simulink model "NichtLinearesModell"  (R2021b)
settings: Solver=ode4  StartTime=0.0  StopTime=250  FixedStep=0.02  RelTol=1e-3
undefined symbols (not defined in the file): AC, BFZ, c, ENV, input_height, input_speed, k_lag, k_p, NickD
settings Model: Creator=falcon  LastModifiedBy=jonih
settings DebuggingCC: UnderSpecifiedDimensionMsg=warning

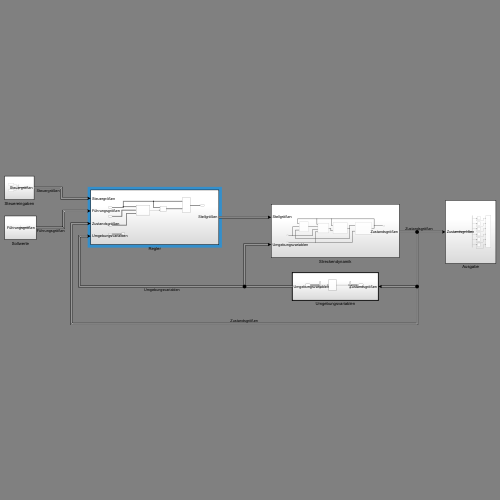
[thumbnail: Simulink's stored preview of the top-level diagram]
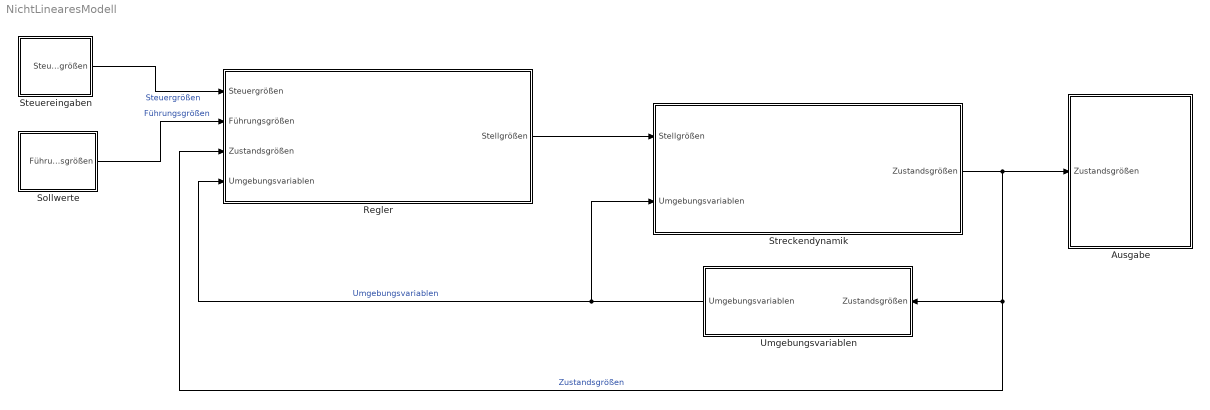
== system NichtLinearesModell ==
  Ausgabe : Subsystem
  Regler : Subsystem
  Sollwerte : Subsystem
  Steuereingaben : Subsystem
  Streckendynamik : Subsystem
  Umgebungsvariablen : Subsystem  TreatAsAtomicUnit=on
  wires:
  Streckendynamik/1(Zustandsgrößen) -> Umgebungsvariablen/1(Zustandsgrößen), Regler/3(Zustandsgrößen), Ausgabe/1(Zustandsgrößen)  "Zustandsgrößen"
  Umgebungsvariablen/1(Umgebungsvariablen) -> Streckendynamik/2(Umgebungsvariablen), Regler/4(Umgebungsvariablen)  "Umgebungsvariablen"
  Sollwerte/1(Führungsgrößen) -> Regler/2(Führungsgrößen)  "Führungsgrößen"
  Steuereingaben/1(Steuergrößen) -> Regler/1(Steuergrößen)  "Steuergrößen"
  Regler/1(Stellgrößen) -> Streckendynamik/1(Stellgrößen)

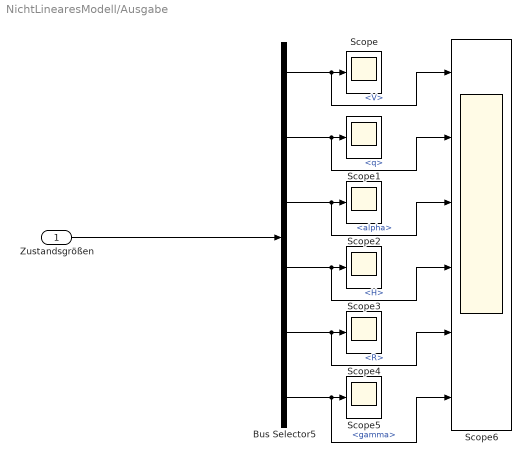
== system NichtLinearesModell/Ausgabe ==
  Zustandsgrößen : Inport
  Bus Selector5 : BusSelector  OutputSignals=V,q,alpha,H,R,gamma
  Scope{,1..5} (6 alike) : Scope
  Scope6 : Scope  NumInputPorts=6
  wires:
  Bus Selector5/4 -> Scope6/4, Scope3/1  "<H>"
  Zustandsgrößen/1 -> Bus Selector5/1
  Bus Selector5/3 -> Scope6/3, Scope2/1  "<alpha>"
  Bus Selector5/6 -> Scope6/6, Scope5/1  "<gamma>"
  Bus Selector5/2 -> Scope6/2, Scope1/1  "<q>"
  Bus Selector5/5 -> Scope6/5, Scope4/1  "<R>"
  Bus Selector5/1 -> Scope6/1, Scope/1  "<V>"

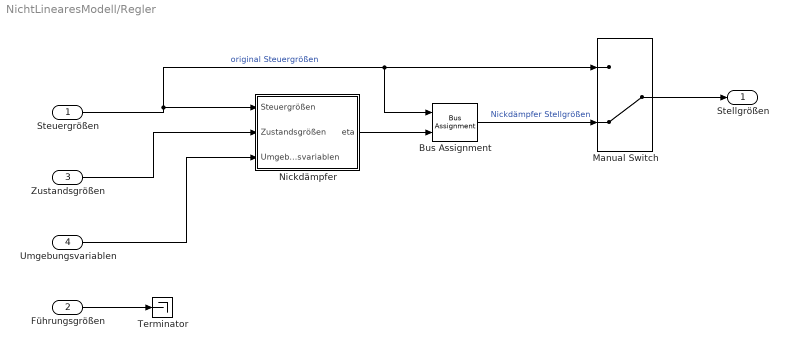
== system NichtLinearesModell/Regler ==
  Steuergrößen : Inport
  Führungsgrößen : Inport  Port=2
  Zustandsgrößen : Inport  Port=3
  Umgebungsvariablen : Inport  Port=4
  Bus Assignment : BusAssignment  AssignedSignals=eta
  Manual Switch : ManualSwitch  CurrentSetting=0
  Nickdämpfer : Subsystem
  Terminator : Terminator
  Stellgrößen : Outport
  wires:
  Steuergrößen/1 -> Nickdämpfer/1(Steuergrößen), Bus Assignment/1, Manual Switch/1  "original Steuergrößen"
  Zustandsgrößen/1 -> Nickdämpfer/2(Zustandsgrößen)
  Nickdämpfer/1(eta) -> Bus Assignment/2
  Führungsgrößen/1 -> Terminator/1
  Bus Assignment/1 -> Manual Switch/2  "Nickdämpfer Stellgrößen"
  Manual Switch/1 -> Stellgrößen/1
  Umgebungsvariablen/1 -> Nickdämpfer/3(Umgebungsvariablen)

== system NichtLinearesModell/Sollwerte ==
  Bus Creator : BusCreator  Inputs=1
  Führungsgrößendummy : Constant  Value=0
  Führungsgrößen : Outport
  wires:
  Führungsgrößendummy/1 -> Bus Creator/1
  Bus Creator/1 -> Führungsgrößen/1  "Führungsgrößen"

== system NichtLinearesModell/Steuereingaben ==
  Bus Creator2 : BusCreator  Inputs=2
  Höhenruderausschlag : Constant  Value=BFZ(8).eta
  Schubdrosselstellung : Constant  Value=BFZ(8).delta
  Steuergrößen : Outport
  wires:
  Höhenruderausschlag/1 -> Bus Creator2/1  "eta"
  Bus Creator2/1 -> Steuergrößen/1  "Steuergrößen"
  Schubdrosselstellung/1 -> Bus Creator2/2  "delta"

== system NichtLinearesModell/Streckendynamik ==
  Stellgrößen : Inport
  Umgebungsvariablen : Inport  Port=2
  Beiwerteberechnung : Subsystem
  Integration : Subsystem
  Kräfte und Momente : Subsystem
  zeitliche Änderung der Zustandsgrößen : Subsystem
  Zustandsgrößen : Outport
  wires:
  Beiwerteberechnung/1(Beiwerte) -> Kräfte und Momente/2(Beiwerte)  "Beiwerte"
  Stellgrößen/1 -> Beiwerteberechnung/2(Steuergrößen), Kräfte und Momente/3(Steuergrößen)  "Stellgrößen"
  Kräfte und Momente/1(Kräfte & Momente) -> zeitliche Änderung der Zustandsgrößen/2(Kräfte & Momente)
  Integration/1(Zustandsgrößen) -> Beiwerteberechnung/1(Zustandsgrößen), Kräfte und Momente/1(Zustandsgrößen), zeitliche Änderung der Zustandsgrößen/1(Zustandsgrößen), Zustandsgrößen/1  "Zustandsgrößen"
  zeitliche Änderung der Zustandsgrößen/1(Änderung der Zustandsgrößen) -> Integration/1(zeitl. Änderung d. Zustandsgrößen), Beiwerteberechnung/3(Änderung der Zustandsgrößen)  "zeitl. Änderung der Zustandsgrößen"
  Umgebungsvariablen/1 -> Kräfte und Momente/4(Umgebungsvariablen), Integration/2(Umgebungsvariablen)  "Umgebungsvariablen"

== system NichtLinearesModell/Umgebungsvariablen ==
  Zustandsgrößen : Inport
  Bus Creator : BusCreator  Inputs=1
  Bus Selector4 : BusSelector  OutputSignals=H
  rho_Berechnung : Subsystem
  Umgebungsvariablen : Outport
  wires:
  Bus Selector4/1 -> rho_Berechnung/1(H)  "<H>"
  rho_Berechnung/1(rho) -> Bus Creator/1  "rho"
  Bus Creator/1 -> Umgebungsvariablen/1
  Zustandsgrößen/1 -> Bus Selector4/1

== system NichtLinearesModell/Regler/Nickdämpfer ==
  Steuergrößen : Inport
  Zustandsgrößen : Inport  Port=2
  Umgebungsvariablen : Inport  Port=3
  Bus Selector : BusSelector  OutputSignals=eta
  Lag-Filter Rückführung : Subsystem
  Manual Switch : ManualSwitch
  Proportionalrückführung : Subsystem
  Sum : Sum  Inputs=+-|
  eta : Outport
  wires:
  Sum/1 -> eta/1  "eta"
  Lag-Filter Rückführung/1(η) -> Manual Switch/1
  Manual Switch/1 -> Sum/2
  Steuergrößen/1 -> Bus Selector/1
  Bus Selector/1 -> Sum/1  "<eta>"
  Proportionalrückführung/1(η) -> Manual Switch/2
  Zustandsgrößen/1 -> Lag-Filter Rückführung/1(Zustandsgrößen), Proportionalrückführung/1(Zustandsgrößen)
  Umgebungsvariablen/1 -> Lag-Filter Rückführung/2(Umgebungsvariablen), Proportionalrückführung/2(Umgebungsvariablen)

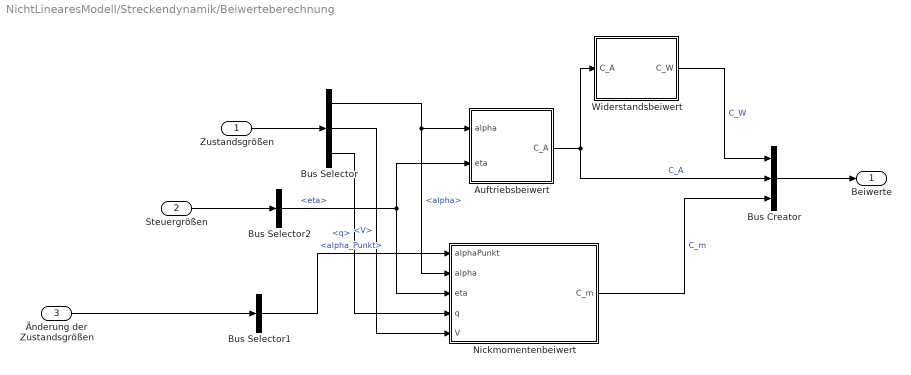
== system NichtLinearesModell/Streckendynamik/Beiwerteberechnung ==
  Zustandsgrößen : Inport
  Steuergrößen : Inport  Port=2
  Änderung der Zustandsgrößen : Inport  Port=3
  Auftriebsbeiwert : Subsystem
  Bus Creator : BusCreator  Inputs=3
  Bus Selector : BusSelector  OutputSignals=alpha,V,q
  Bus Selector1 : BusSelector  OutputSignals=alpha_Punkt
  Bus Selector2 : BusSelector  OutputSignals=eta
  Nickmomentenbeiwert : Subsystem
  Widerstandsbeiwert : Subsystem
  Beiwerte : Outport
  wires:
  Nickmomentenbeiwert/1(C_m) -> Bus Creator/3  "C_m"
  Auftriebsbeiwert/1(C_A) -> Bus Creator/2, Widerstandsbeiwert/1(C_A)  "C_A"
  Bus Selector/1 -> Auftriebsbeiwert/1(alpha), Nickmomentenbeiwert/2(alpha)  "<alpha>"
  Bus Creator/1 -> Beiwerte/1
  Widerstandsbeiwert/1(C_W) -> Bus Creator/1  "C_W"
  Zustandsgrößen/1 -> Bus Selector/1
  Änderung der Zustandsgrößen/1 -> Bus Selector1/1
  Bus Selector1/1 -> Nickmomentenbeiwert/1(alphaPunkt)  "<alpha_Punkt>"
  Bus Selector/2 -> Nickmomentenbeiwert/5(V)  "<V>"
  Bus Selector/3 -> Nickmomentenbeiwert/4(q)  "<q>"
  Steuergrößen/1 -> Bus Selector2/1
  Bus Selector2/1 -> Nickmomentenbeiwert/3(eta), Auftriebsbeiwert/2(eta)  "<eta>"

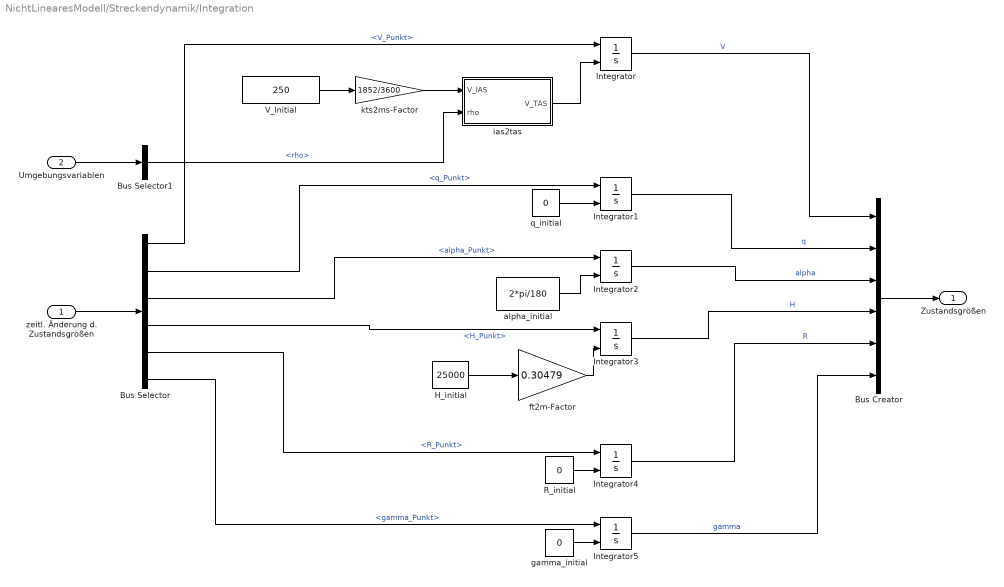
== system NichtLinearesModell/Streckendynamik/Integration ==
  zeitl. Änderung d. Zustandsgrößen : Inport
  Umgebungsvariablen : Inport  Port=2
  Bus Creator : BusCreator  Inputs=6
  Bus Selector : BusSelector  OutputSignals=V_Punkt,q_Punkt,alpha_Punkt,H_Punkt,R_Punkt,gamma_Punkt
  Bus Selector1 : BusSelector  OutputSignals=rho
  H_initial : Constant  Value=25000
  Integrator{,1..5} (6 alike) : Integrator  InitialConditionSource=external
  R_initial : Constant  Value=0
  V_Initial : Constant  Value=250
  alpha_initial : Constant  Value=2*pi/180
  ft2m-Factor : Gain  Gain=0.30479
  gamma_initial : Constant  Value=0
  ias2tas : Subsystem
  kts2ms-Factor : Gain  Gain=1852/3600
  q_initial : Constant  Value=0
  Zustandsgrößen : Outport
  wires:
  Bus Selector/5 -> Integrator4/1  "<R_Punkt>"
  gamma_initial/1 -> Integrator5/2
  Bus Selector/3 -> Integrator2/1  "<alpha_Punkt>"
  Integrator2/1 -> Bus Creator/3  "alpha"
  alpha_initial/1 -> Integrator2/2
  Integrator1/1 -> Bus Creator/2  "q"
  Integrator4/1 -> Bus Creator/5  "R"
  Integrator3/1 -> Bus Creator/4  "H"
  Integrator5/1 -> Bus Creator/6  "gamma"
  ias2tas/1(V_TAS) -> Integrator/2
  R_initial/1 -> Integrator4/2
  q_initial/1 -> Integrator1/2
  Bus Selector/6 -> Integrator5/1  "<gamma_Punkt>"
  Bus Selector/2 -> Integrator1/1  "<q_Punkt>"
  Bus Selector/4 -> Integrator3/1  "<H_Punkt>"
  Integrator/1 -> Bus Creator/1  "V"
  Bus Selector/1 -> Integrator/1  "<V_Punkt>"
  V_Initial/1 -> kts2ms-Factor/1
  kts2ms-Factor/1 -> ias2tas/1(V_IAS)
  Bus Selector1/1 -> ias2tas/2(rho)  "<rho>"
  H_initial/1 -> ft2m-Factor/1
  ft2m-Factor/1 -> Integrator3/2
  Bus Creator/1 -> Zustandsgrößen/1
  zeitl. Änderung d. Zustandsgrößen/1 -> Bus Selector/1
  Umgebungsvariablen/1 -> Bus Selector1/1

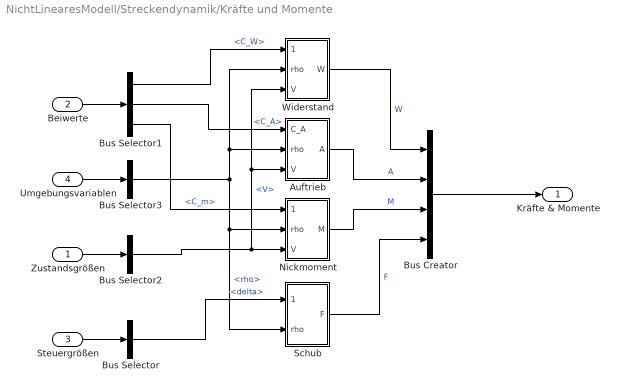
== system NichtLinearesModell/Streckendynamik/Kräfte und Momente ==
  Zustandsgrößen : Inport
  Beiwerte : Inport  Port=2
  Steuergrößen : Inport  Port=3
  Umgebungsvariablen : Inport  Port=4
  Auftrieb : Subsystem
  Bus Creator : BusCreator  Inputs=4
  Bus Selector : BusSelector  OutputSignals=delta
  Bus Selector1 : BusSelector  OutputSignals=C_W,C_A,C_m
  Bus Selector2 : BusSelector  OutputSignals=V
  Bus Selector3 : BusSelector  OutputSignals=rho
  Nickmoment : Subsystem
  Schub : Subsystem
  Widerstand : Subsystem
  Kräfte & Momente : Outport
  wires:
  Widerstand/1(W) -> Bus Creator/1  "W"
  Auftrieb/1(A) -> Bus Creator/2  "A"
  Nickmoment/1(M) -> Bus Creator/3  "M"
  Schub/1(F) -> Bus Creator/4  "F"
  Bus Creator/1 -> Kräfte & Momente/1
  Beiwerte/1 -> Bus Selector1/1
  Zustandsgrößen/1 -> Bus Selector2/1
  Steuergrößen/1 -> Bus Selector/1
  Bus Selector/1 -> Schub/1(delta)  "<delta>"
  Bus Selector1/2 -> Auftrieb/1(C_A)  "<C_A>"
  Bus Selector1/1 -> Widerstand/1(C_W)  "<C_W>"
  Bus Selector1/3 -> Nickmoment/1(C_m)  "<C_m>"
  Umgebungsvariablen/1 -> Bus Selector3/1
  Bus Selector3/1 -> Nickmoment/2(rho), Schub/2(rho), Auftrieb/2(rho), Widerstand/2(rho)  "<rho>"
  Bus Selector2/1 -> Nickmoment/3(V), Auftrieb/3(V), Widerstand/3(V)  "<V>"

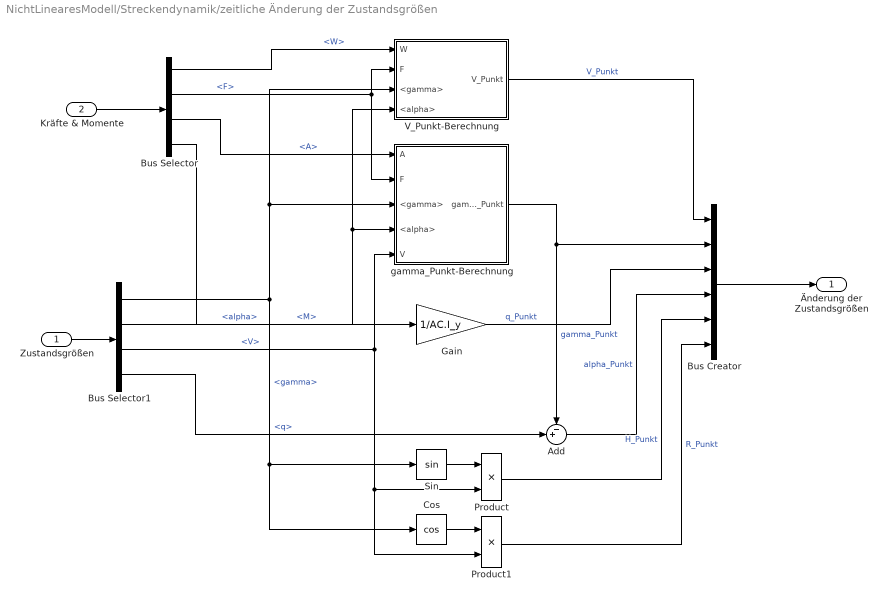
== system NichtLinearesModell/Streckendynamik/zeitliche Änderung der Zustandsgrößen ==
  Zustandsgrößen : Inport
  Kräfte & Momente : Inport  Port=2
  Add : Sum  Inputs=-+|
  Bus Creator : BusCreator  Inputs=6
  Bus Selector : BusSelector  OutputSignals=W,F,A,M
  Bus Selector1 : BusSelector  OutputSignals=gamma,alpha,V,q
  Cos : Trigonometry  Operator=cos
  Gain : Gain  Gain=1/AC.I_y
  Product : Product
  Product1 : Product
  Sin : Trigonometry
  V_Punkt-Berechnung : Subsystem
  gamma_Punkt-Berechnung : Subsystem
  Änderung der Zustandsgrößen : Outport
  wires:
  V_Punkt-Berechnung/1(V_Punkt) -> Bus Creator/1  "V_Punkt"
  Sin/1 -> Product/1
  Add/1 -> Bus Creator/4  "alpha_Punkt"
  Bus Selector/3 -> gamma_Punkt-Berechnung/1(A)  "<A>"
  gamma_Punkt-Berechnung/1(gamma_Punkt) -> Bus Creator/2, Add/1  "gamma_Punkt"
  Gain/1 -> Bus Creator/3  "q_Punkt"
  Bus Selector/4 -> Gain/1  "<M>"
  Cos/1 -> Product1/1
  Bus Selector/1 -> V_Punkt-Berechnung/1(W)  "<W>"
  Bus Selector1/2 -> gamma_Punkt-Berechnung/4(<alpha>), V_Punkt-Berechnung/4(<alpha>)  "<alpha>"
  Product/1 -> Bus Creator/5  "H_Punkt"
  Bus Selector1/1 -> Sin/1, Cos/1, V_Punkt-Berechnung/3(<gamma>), gamma_Punkt-Berechnung/3(<gamma>)  "<gamma>"
  Bus Selector1/3 -> Product1/2, Product/2, gamma_Punkt-Berechnung/5(V)  "<V>"
  Product1/1 -> Bus Creator/6  "R_Punkt"
  Bus Selector/2 -> gamma_Punkt-Berechnung/2(F), V_Punkt-Berechnung/2(F)  "<F>"
  Bus Selector1/4 -> Add/2  "<q>"
  Zustandsgrößen/1 -> Bus Selector1/1
  Kräfte & Momente/1 -> Bus Selector/1
  Bus Creator/1 -> Änderung der Zustandsgrößen/1

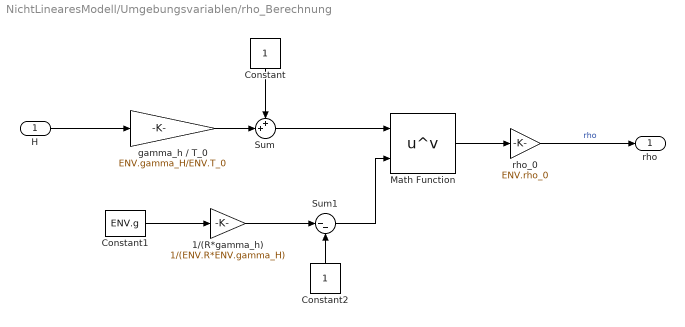
== system NichtLinearesModell/Umgebungsvariablen/rho_Berechnung ==
  H : Inport
  1/(R*gamma_h) : Gain  Gain=1/(ENV.R*ENV.gamma_H)
  Constant : Constant
  Constant1 : Constant  Value=ENV.g
  Constant2 : Constant
  Math Function : Math  Operator=pow  SaturateOnIntegerOverflow=on
  Sum : Sum  Inputs=++|
  Sum1 : Sum  Inputs=|--
  gamma_h / T_0 : Gain  Gain=ENV.gamma_H/ENV.T_0
  rho_0 : Gain  Gain=ENV.rho_0
  rho : Outport
  wires:
  1/(R*gamma_h)/1 -> Sum1/1
  gamma_h / T_0/1 -> Sum/2
  Constant1/1 -> 1/(R*gamma_h)/1
  Sum/1 -> Math Function/1
  H/1 -> gamma_h / T_0/1
  Sum1/1 -> Math Function/2
  rho_0/1 -> rho/1  "rho"
  Constant2/1 -> Sum1/2
  Math Function/1 -> rho_0/1
  Constant/1 -> Sum/1

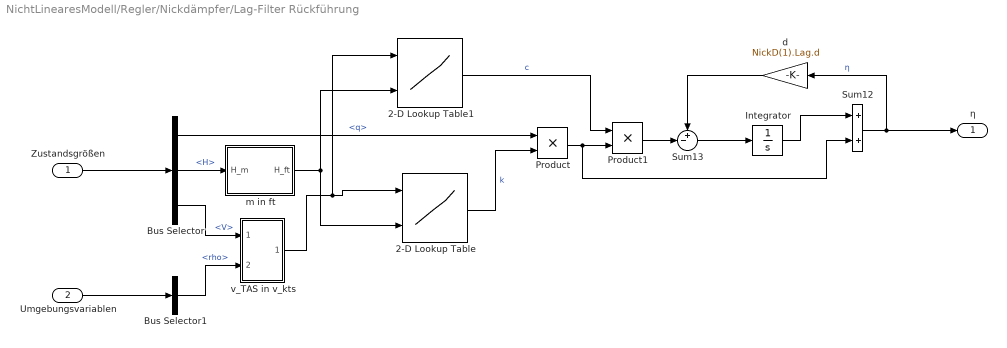
== system NichtLinearesModell/Regler/Nickdämpfer/Lag-Filter Rückführung ==
  Zustandsgrößen : Inport
  Umgebungsvariablen : Inport  Port=2
  2-D Lookup Table : Lookup_n-D  BreakpointsForDimension1=input_speed  BreakpointsForDimension2=input_height  Table=reshape(k_lag,[length(input_speed),length(input_height)])  InternalRulePriority=Speed  RndMeth=Simplest  InputSameDT=on
      settings: InputPortMap=u0,u1
  2-D Lookup Table1 : Lookup_n-D  BreakpointsForDimension1=input_speed  BreakpointsForDimension2=input_height  Table=reshape(c,[length(input_speed),length(input_height)])  InternalRulePriority=Speed  RndMeth=Simplest  InputSameDT=on
      settings: InputPortMap=u0,u1
  Bus Selector : BusSelector  OutputSignals=q,H,V
  Bus Selector1 : BusSelector  OutputSignals=rho
  Integrator : Integrator
  Product : Product
  Product1 : Product
  Sum12 : Sum
  Sum13 : Sum  Inputs=+-|
  d : Gain  Gain=NickD(1).Lag.d
  m in ft : Subsystem
  v_TAS in v_kts : Subsystem
  η : Outport
  wires:
  d/1 -> Sum13/1
  Sum13/1 -> Integrator/1
  Sum12/1 -> η/1, d/1  "η"
  Integrator/1 -> Sum12/1
  Product1/1 -> Sum13/2
  Zustandsgrößen/1 -> Bus Selector/1
  Bus Selector/1 -> Product/1  "<q>"
  Product/1 -> Product1/2, Sum12/2
  Bus Selector/3 -> v_TAS in v_kts/1(V_TAS)  "<V>"
  Umgebungsvariablen/1 -> Bus Selector1/1
  Bus Selector1/1 -> v_TAS in v_kts/2(rho)  "<rho>"
  Bus Selector/2 -> m in ft/1(H_m)  "<H>"
  2-D Lookup Table1/1 -> Product1/1  "c"
  2-D Lookup Table/1 -> Product/2  "k"
  m in ft/1(H_ft) -> 2-D Lookup Table/2, 2-D Lookup Table1/2
  v_TAS in v_kts/1(v_kts) -> 2-D Lookup Table1/1, 2-D Lookup Table/1

== system NichtLinearesModell/Regler/Nickdämpfer/Proportionalrückführung ==
  Zustandsgrößen : Inport
  Umgebungsvariablen : Inport  Port=2
  2-D Lookup Table : Lookup_n-D  BreakpointsForDimension1=input_speed  BreakpointsForDimension2=input_height  Table=reshape(k_p,[length(input_speed),length(input_height)])  InternalRulePriority=Speed  RndMeth=Simplest  InputSameDT=on
      settings: InputPortMap=u0,u1
  Bus Selector : BusSelector  OutputSignals=q,V,H
  Bus Selector2 : BusSelector  OutputSignals=rho
  Product : Product
  m in ft : Subsystem
  v_TAS in v_kts : Subsystem
  η : Outport
  wires:
  Product/1 -> η/1  "eta"
  Zustandsgrößen/1 -> Bus Selector/1
  Bus Selector/1 -> Product/1  "<q>"
  2-D Lookup Table/1 -> Product/2  "k_p"
  Umgebungsvariablen/1 -> Bus Selector2/1
  Bus Selector2/1 -> v_TAS in v_kts/2(rho)  "<rho>"
  Bus Selector/3 -> m in ft/1(H_m)  "<H>"
  Bus Selector/2 -> v_TAS in v_kts/1(V_TAS)  "<V>"
  m in ft/1(H_ft) -> 2-D Lookup Table/2
  v_TAS in v_kts/1(v_kts) -> 2-D Lookup Table/1

== system NichtLinearesModell/Streckendynamik/Beiwerteberechnung/Auftriebsbeiwert ==
  alpha : Inport
  eta : Inport  Port=2
  Constant1 : Constant  Value=AC.C_A_Alpha0Eta0
  Gain : Gain  Gain=AC.C_A_Eta
  Gain2 : Gain  Gain=AC.C_A_Alpha
  Sum : Sum  Inputs=+++
  C_A : Outport
  wires:
  Constant1/1 -> Sum/1
  Gain2/1 -> Sum/2
  eta/1 -> Gain/1
  Gain/1 -> Sum/3
  alpha/1 -> Gain2/1
  Sum/1 -> C_A/1  "C_A"

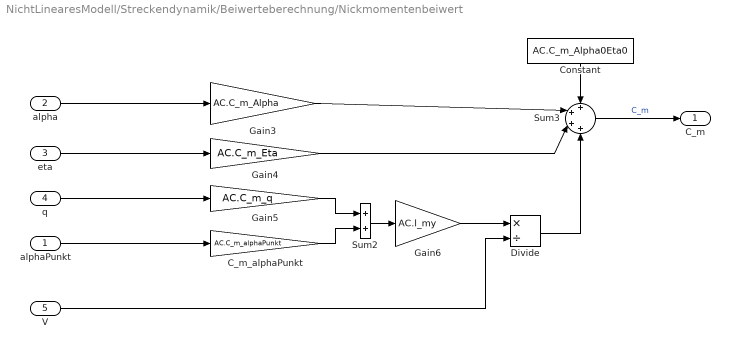
== system NichtLinearesModell/Streckendynamik/Beiwerteberechnung/Nickmomentenbeiwert ==
  alphaPunkt : Inport
  alpha : Inport  Port=2
  eta : Inport  Port=3
  q : Inport  Port=4
  V : Inport  Port=5
  C_m_alphaPunkt : Gain  Gain=AC.C_m_alphaPunkt
  Constant : Constant  Value=AC.C_m_Alpha0Eta0
  Divide : Product  Inputs=*/
  Gain3 : Gain  Gain=AC.C_m_Alpha
  Gain4 : Gain  Gain=AC.C_m_Eta
  Gain5 : Gain  Gain=AC.C_m_q
  Gain6 : Gain  Gain=AC.l_my
  Sum2 : Sum
  Sum3 : Sum  Inputs=++++
  C_m : Outport
  wires:
  Gain3/1 -> Sum3/2
  Divide/1 -> Sum3/4
  V/1 -> Divide/2
  C_m_alphaPunkt/1 -> Sum2/2
  Gain4/1 -> Sum3/3
  q/1 -> Gain5/1
  Constant/1 -> Sum3/1
  Gain6/1 -> Divide/1
  Gain5/1 -> Sum2/1
  alpha/1 -> Gain3/1
  Sum2/1 -> Gain6/1
  Sum3/1 -> C_m/1  "C_m"
  eta/1 -> Gain4/1
  alphaPunkt/1 -> C_m_alphaPunkt/1

== system NichtLinearesModell/Streckendynamik/Beiwerteberechnung/Widerstandsbeiwert ==
  C_A : Inport
  Constant2 : Constant  Value=AC.C_W0
  Gain1 : Gain  Gain=AC.k
  Square : Math  Operator=square  SaturateOnIntegerOverflow=on
  Sum1 : Sum  Inputs=|++
  C_W : Outport
  wires:
  Constant2/1 -> Sum1/1
  Sum1/1 -> C_W/1  "C_W"
  Square/1 -> Gain1/1
  C_A/1 -> Square/1
  Gain1/1 -> Sum1/2

== system NichtLinearesModell/Streckendynamik/Integration/ias2tas ==
  V_IAS : Inport
  rho : Inport  Port=2
  Constant : Constant  Value=1.225
  Divide : Product  Inputs=*/
  Product : Product
  Sqrt : Sqrt  SaturateOnIntegerOverflow=on
  V_TAS : Outport
  wires:
  Product/1 -> V_TAS/1
  V_IAS/1 -> Product/1
  Constant/1 -> Divide/1
  rho/1 -> Divide/2
  Divide/1 -> Sqrt/1
  Sqrt/1 -> Product/2

== system NichtLinearesModell/Streckendynamik/Kräfte und Momente/Auftrieb ==
  C_A : Inport
  rho : Inport  Port=2
  V : Inport  Port=3
  Gain : Gain  Gain=0.5
  Gain1 : Gain  Gain=AC.S
  Product : Product  Inputs=3
  Square : Math  Operator=square  SaturateOnIntegerOverflow=on
  A : Outport
  wires:
  rho/1 -> Gain/1
  Square/1 -> Product/3
  Product/1 -> Gain1/1
  Gain1/1 -> A/1  "A"
  V/1 -> Square/1
  Gain/1 -> Product/2
  C_A/1 -> Product/1

== system NichtLinearesModell/Streckendynamik/Kräfte und Momente/Nickmoment ==
  C_m : Inport
  rho : Inport  Port=2
  V : Inport  Port=3
  Gain : Gain  Gain=0.5
  Gain1 : Gain  Gain=AC.S
  Gain2 : Gain  Gain=AC.l_my
  Product : Product  Inputs=3
  Square : Math  Operator=square  SaturateOnIntegerOverflow=on
  M : Outport
  wires:
  rho/1 -> Gain/1
  Square/1 -> Product/3
  Product/1 -> Gain1/1
  Gain1/1 -> Gain2/1
  V/1 -> Square/1
  Gain/1 -> Product/2
  C_m/1 -> Product/1
  Gain2/1 -> M/1

== system NichtLinearesModell/Streckendynamik/Kräfte und Momente/Schub ==
  delta : Inport
  rho : Inport  Port=2
  Constant : Constant  Value=AC.n_rho
  Gain : Gain  Gain=AC.F_TBPmax
  Math Function : Math  Operator=pow  SaturateOnIntegerOverflow=on
  Multiply : Gain  Gain=1/AC.rho_TBP
  Product : Product
  F : Outport
  wires:
  rho/1 -> Multiply/1
  Constant/1 -> Math Function/2
  Product/1 -> F/1  "F"
  Math Function/1 -> Product/2
  Gain/1 -> Product/1
  Multiply/1 -> Math Function/1
  delta/1 -> Gain/1

== system NichtLinearesModell/Streckendynamik/Kräfte und Momente/Widerstand ==
  C_W : Inport
  rho : Inport  Port=2
  V : Inport  Port=3
  Gain : Gain  Gain=0.5
  Gain1 : Gain  Gain=AC.S
  Product : Product  Inputs=3
  Square : Math  Operator=square  SaturateOnIntegerOverflow=on
  W : Outport
  wires:
  rho/1 -> Gain/1
  Square/1 -> Product/3
  Product/1 -> Gain1/1
  Gain1/1 -> W/1  "W"
  V/1 -> Square/1
  Gain/1 -> Product/2
  C_W/1 -> Product/1

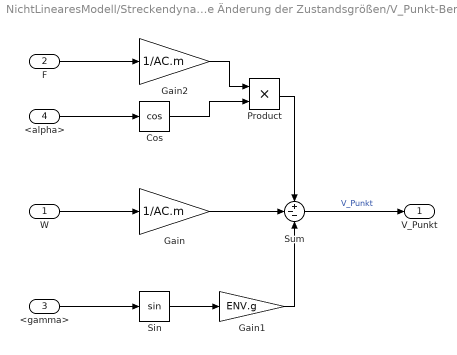
== system NichtLinearesModell/Streckendynamik/zeitliche Änderung der Zustandsgrößen/V_Punkt-Berechnung ==
  W : Inport
  F : Inport  Port=2
  <gamma> : Inport  Port=3
  <alpha> : Inport  Port=4
  Cos : Trigonometry  Operator=cos
  Gain : Gain  Gain=1/AC.m
  Gain1 : Gain  Gain=ENV.g
  Gain2 : Gain  Gain=1/AC.m
  Product : Product
  Sin : Trigonometry
  Sum : Sum  Inputs=+--
  V_Punkt : Outport
  wires:
  Gain1/1 -> Sum/3
  Gain2/1 -> Product/1
  <gamma>/1 -> Sin/1
  Product/1 -> Sum/1
  W/1 -> Gain/1
  Sin/1 -> Gain1/1
  Sum/1 -> V_Punkt/1  "V_Punkt"
  Cos/1 -> Product/2
  <alpha>/1 -> Cos/1
  F/1 -> Gain2/1
  Gain/1 -> Sum/2

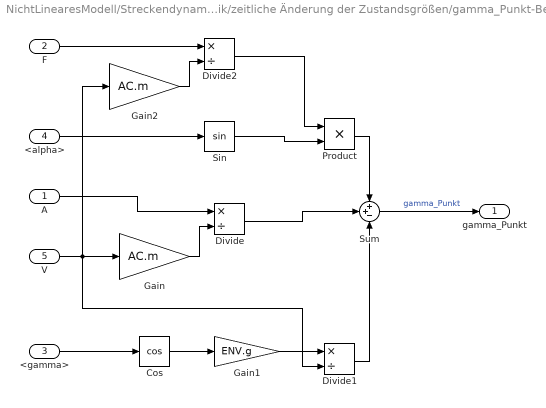
== system NichtLinearesModell/Streckendynamik/zeitliche Änderung der Zustandsgrößen/gamma_Punkt-Berechnung ==
  A : Inport
  F : Inport  Port=2
  <gamma> : Inport  Port=3
  <alpha> : Inport  Port=4
  V : Inport  Port=5
  Cos : Trigonometry  Operator=cos
  Divide : Product  Inputs=*/
  Divide1 : Product  Inputs=*/
  Divide2 : Product  Inputs=*/
  Gain : Gain  Gain=AC.m
  Gain1 : Gain  Gain=ENV.g
  Gain2 : Gain  Gain=AC.m
  Product : Product
  Sin : Trigonometry
  Sum : Sum  Inputs=++-
  gamma_Punkt : Outport
  wires:
  Divide2/1 -> Product/1
  <gamma>/1 -> Cos/1
  Product/1 -> Sum/1
  Cos/1 -> Gain1/1
  Sum/1 -> gamma_Punkt/1  "gamma_Punkt"
  Sin/1 -> Product/2
  F/1 -> Divide2/1
  <alpha>/1 -> Sin/1
  V/1 -> Gain2/1, Divide1/2, Gain/1
  Gain/1 -> Divide/2
  A/1 -> Divide/1
  Divide/1 -> Sum/2
  Gain1/1 -> Divide1/1
  Divide1/1 -> Sum/3
  Gain2/1 -> Divide2/2

== system NichtLinearesModell/Regler/Nickdämpfer/Lag-Filter Rückführung/m in ft ==
  H_m : Inport
  m2ft : Gain  Gain=1/0.30479
  H_ft : Outport
  wires:
  m2ft/1 -> H_ft/1
  H_m/1 -> m2ft/1

== system NichtLinearesModell/Regler/Nickdämpfer/Lag-Filter Rückführung/v_TAS in v_kts ==
  V_TAS : Inport
  rho : Inport  Port=2
  ms2kts : Subsystem
  tas2ias : Subsystem
  v_kts : Outport
  wires:
  rho/1 -> tas2ias/2(rho)
  tas2ias/1(v_IAS) -> ms2kts/1(v_ms)
  ms2kts/1(v_kts) -> v_kts/1
  V_TAS/1 -> tas2ias/1(V_TAS)

== system NichtLinearesModell/Regler/Nickdämpfer/Proportionalrückführung/m in ft ==
  H_m : Inport
  m2ft : Gain  Gain=1/0.30479
  H_ft : Outport
  wires:
  m2ft/1 -> H_ft/1
  H_m/1 -> m2ft/1

== system NichtLinearesModell/Regler/Nickdämpfer/Proportionalrückführung/v_TAS in v_kts ==
  V_TAS : Inport
  rho : Inport  Port=2
  ms2kts : Subsystem
  tas2ias : Subsystem
  v_kts : Outport
  wires:
  rho/1 -> tas2ias/2(rho)
  tas2ias/1(v_IAS) -> ms2kts/1(v_ms)
  ms2kts/1(v_kts) -> v_kts/1
  V_TAS/1 -> tas2ias/1(V_TAS)

== system NichtLinearesModell/Regler/Nickdämpfer/Lag-Filter Rückführung/v_TAS in v_kts/ms2kts ==
  v_ms : Inport
  Gain : Gain  Gain=3600/1852
  v_kts : Outport
  wires:
  Gain/1 -> v_kts/1
  v_ms/1 -> Gain/1

== system NichtLinearesModell/Regler/Nickdämpfer/Lag-Filter Rückführung/v_TAS in v_kts/tas2ias ==
  V_TAS : Inport
  rho : Inport  Port=2
  Constant : Constant  Value=1.225
  Divide : Product  Inputs=*/
  Divide1 : Product  Inputs=*/
  Sqrt : Sqrt  SaturateOnIntegerOverflow=on
  v_IAS : Outport
  wires:
  Constant/1 -> Divide/1
  rho/1 -> Divide/2
  Divide/1 -> Sqrt/1
  V_TAS/1 -> Divide1/1
  Sqrt/1 -> Divide1/2
  Divide1/1 -> v_IAS/1

== system NichtLinearesModell/Regler/Nickdämpfer/Proportionalrückführung/v_TAS in v_kts/ms2kts ==
  v_ms : Inport
  Gain : Gain  Gain=3600/1852
  v_kts : Outport
  wires:
  Gain/1 -> v_kts/1
  v_ms/1 -> Gain/1

== system NichtLinearesModell/Regler/Nickdämpfer/Proportionalrückführung/v_TAS in v_kts/tas2ias ==
  V_TAS : Inport
  rho : Inport  Port=2
  Constant : Constant  Value=1.225
  Divide : Product  Inputs=*/
  Divide1 : Product  Inputs=*/
  Sqrt : Sqrt  SaturateOnIntegerOverflow=on
  v_IAS : Outport
  wires:
  Constant/1 -> Divide/1
  rho/1 -> Divide/2
  Divide/1 -> Sqrt/1
  V_TAS/1 -> Divide1/1
  Sqrt/1 -> Divide1/2
  Divide1/1 -> v_IAS/1
